simulink model "phasenoise_sim"  (Simulink 6.0)
settings: Solver=ode45  StartTime=0.0  StopTime=10  RelTol=1e-3
undefined symbols (not defined in the file or in its folder): slcm
libraries: commsink2 x2, commdigbbndam2 x2, commchan2 x1, commrflib2 x1, commrandsrc2 x1
CloseFcn:
  | clear phnoiseSigsOut
settings Model: Creator=mikem  LastModifiedBy=arodrigu
settings DataIOCC: SaveOutput=off  SaveTime=off  SignalLoggingName=phnoiseSigsOut
settings OptimizationCC: BlockReduction=off  BooleanDataType=off
settings DebuggingCC: CheckExecutionContextPreStartOutputMsg=on  CheckExecutionContextRuntimeOutputMsg=on  SolverPrmCheckMsg=none  InheritedTsInSrcMsg=none
settings HardwareCC: TargetUnknown=on
settings ModelReferenceCC: UpdateModelReferenceTargets=IfOutOfDate

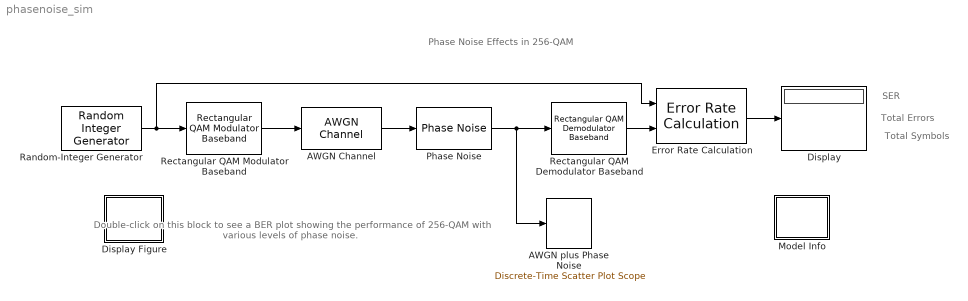
== system phasenoise_sim ==
  note: Phase Noise Effects in 256-QAM
  note: Double-click on this block to see a BER plot
      | showing the performance of 256-QAM
      | with various levels of phase noise.
  note: SER
  note: Total Errors
  note: Total Symbols
  AWGN Channel : commchan2/AWGN Channel  seed=54321  noiseMode="Signal to noise ratio  (Es/No)"  EbNodB=10  EsNodB=40  SNRdB=10  bitsPerSym=1  Ps=1  Tsym=.001  variance=1
  AWGN plus Phase Noise : commsink2/Discrete-Time Scatter Plot Scope  Tag=ScatterPlot  sampPerSymb=1  offsetEye=0  numTraces=2500  numNewFrames=300  LineMarkers=.  LineColors=b  fading=on  render=on  AxisGrid=on  xMin=-1.5  xMax=1.5  yMin=-1.5  yMax=1.5  inphaseLabel=In-phase Amplitude  quadratureLabel=Quadrature Amplitude  openScopeAtSimStart=on  FrameNumber=off  FigPos=[384 243 576 576]  figTitle=Scatter Plot  numLinesMax=8  block_type_=scatter
  Display : Display
  Display Figure : Subsystem  PropExecContextAcrossSSBoundary=on
      settings: OpenFcn=openfig phasenoise256qam.fig;
      mask Type: Display Figure
      mask Display: disp('Display\nFigure');
  Error Rate Calculation : commsink2/Error Rate Calculation  N=0  st_delay=0  cp_mode=Entire frame  subframe=[]  PMode=Port  WsName=ErrorVec  RsMode2=off  stop=off  numErr=100  maxBits=1e6
  Model Info : Subsystem  LoadFcn=slcm LoadBlock;  InitFcn=slcm('UpdateAllCMBlocksInThisModelInit')  PropExecContextAcrossSSBoundary=on  mask(CMBlock){InitialSaveTempField=, InitialBlockCM=none, BlockCM=none, Frame=on, SaveTempField=, DisplayStringWithTags=Info, MaskDisplayString=Info, HorizontalTextAlignment=Center, LeftAlignmentValue=0.5, SourceBlockDiagram=phasenoise_sim, TagMaxNumber=20, CMTag1=, CMTag2=, CMTag3=, CMTag4=, CMTag5=, CMTag6=, CMTag7=, CMTag8=, CMTag9=, CMTag10=, CMTag11=, CMTag12=, CMTag13=, CMTag14=, CMTag15=, CMTag16=, CMTag17=, CMTag18=, CMTag19=, CMTag20=}
      mask help: This block allows revision control information to be displayed within the model.
      settings: CopyFcn=slcm CopyBlock;  DeleteFcn=slcm Cancel;  PostSaveFcn=slcm('UpdateAllCMBlocksInThisModel')  NameChangeFcn=slcm Rename;  OpenFcn=commdemohelp;
      mask Display: text(str2num(LeftAlignmentValue), 0.5, MaskDisplayString, 'HorizontalAlignment', HorizontalTextAlignment)
  Phase Noise : commrflib2/Phase Noise  PhNs=-66  Fo=200  seed=2137
  Random-Integer Generator : commrandsrc2/Random Integer Generator  mul=256  seed=12345  Ts=.001  frameBased=on  sampPerFrame=500  orient=off
  Rectangular QAM Demodulator Baseband : commdigbbndam2/Rectangular QAM Demodulator Baseband  M=256  OutType=Integer  Dec=Binary  PowType=Average Power  MinDist=2  AvgPow=1  PeakPow=1  Ph=0  numSamp=1
  Rectangular QAM Modulator Baseband : commdigbbndam2/Rectangular QAM Modulator Baseband  M=256  InType=Integer  Enc=Binary  PowType=Average Power  MinDist=2  AvgPow=1  PeakPow=1  Ph=0  numSamp=1
  wires:
  AWGN Channel/1 -> Phase Noise/1
  Rectangular QAM Modulator Baseband/1 -> AWGN Channel/1
  Random-Integer Generator/1 -> Rectangular QAM Modulator Baseband/1, Error Rate Calculation/1
  Phase Noise/1 -> Rectangular QAM Demodulator Baseband/1, AWGN plus Phase Noise/1
  Rectangular QAM Demodulator Baseband/1 -> Error Rate Calculation/2
  Error Rate Calculation/1 -> Display/1

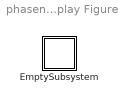
== system phasenoise_sim/Display Figure ==
  EmptySubsystem : Subsystem  PropExecContextAcrossSSBoundary=on

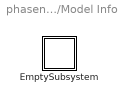
== system phasenoise_sim/Model Info ==
  EmptySubsystem : Subsystem  PropExecContextAcrossSSBoundary=on

== system phasenoise_sim/Display Figure/EmptySubsystem ==

== system phasenoise_sim/Model Info/EmptySubsystem ==
